simulink model "TPMCC_MCLV2_dsPIC33EP256MC506_V0_1"  (R2017a)
settings: Solver=FixedStepDiscrete  StartTime=0.0  StopTime=inf  FixedStep=Ts  RelTol=1e-3  EnableMultiTasking=on
values from neighbouring files (symbols this model uses):
  a = [1.0000   -0.5095]    [InitTPV0.m]
  b = [0.2452    0.2452]    [InitTPV0.m]
  Lignes = 250*4    (= 1000)    [InitTPV0.m]
  PWMmax = 3199    [InitTPV0.m]
  Tm = 0.5e-6    (= 5e-07)    [InitTPV0.m]
  TPWM = 1/FPWM    (= 5e-05)    [InitTPV0.m]
  Ts = 1e-4    (= 0.0001)    [InitTPV0.m]
  Vdc = 24    [InitTPV0.m]
undefined symbols (not defined in the file or in its folder): A4, A8, C5, C6, F1, P20, P24, P53, P54, P97, Pin, Timer
libraries: MCHP_Blockset x23, simulink x5
settings Model: Creator=rdelpoux  LastModifiedBy=rdelpoux
settings OptimizationCC: DefaultParameterBehavior=Inlined  DefaultUnderspecifiedDataType=single  BooleansAsBitfields=on  PassReuseOutputArgsAs=Individual arguments
settings DebuggingCC: ParameterOverflowMsg=warning  ParameterTunabilityLossMsg=error
settings HardwareCC: ProdBitPerInt=16  ProdBitPerPointer=16  ProdBitPerSizeT=16  ProdBitPerPtrDiffT=16  ProdLargestAtomicInteger=Integer  ProdLargestAtomicFloat=None  ProdWordSize=16  ProdHWDeviceType=Generic->Custom
settings ModelReferenceCC: ModelReferenceNumInstancesAllowed=Single
settings SFSimCC: MATLABDynamicMemAlloc=off
settings RTWCC: SystemTargetFile=MCHP_dsPIC_stf.tlc  TemplateMakefile=MCHP_dsPIC.tmf  Description=Microchip Embedded Target PIC24 dsPIC30 dsPIC33 (real-time)  GenerateReport=on  CustomSource=code.c  IncludeHyperlinkInReport=on  LaunchReport=on  GenerateTraceInfo=on  GenerateTraceReport=on  GenerateTraceReportSl=on  GenerateTraceReportSf=on  GenerateTraceReportEml=on
settings CodeAppCC: ForceParamTrailComments=on  IgnoreCustomStorageClasses=off  MaxIdLength=255  OperatorAnnotations=on  SimulinkDataObjDesc=on  SFDataObjDesc=on  MATLABFcnDesc=on  InsertBlockDesc=on  MATLABSourceComments=on
settings STFCustomTargetCC: TargetLibSuffix=_lib.a  MultiwordLength=256  IncludeMdlTerminateFcn=off  CombineOutputUpdateFcns=on  CombineSignalStateStructs=on  SuppressErrorStatus=on  ERTCustomFileBanners=on  SupportContinuousTime=off  RemoveResetFunc=on  MATLABClassNameForMDSCustomization=Simulink.SoftwareTarget.ERTCustomization  GRTInterface=off  SystemTargetFile=MCHP_dsPIC_stf.tlc
settings ERTTargetCC: TargetLibSuffix=_lib.a  ParMdlRefBuildCompliant=off  CompOptLevelCompliant=off  ConcurrentExecutionCompliant=off  IncludeMdlTerminateFcn=off  CombineSignalStateStructs=on  SuppressErrorStatus=on  ERTFirstTimeCompliant=off  SupportNonInlinedSFcns=on  ModelStepFunctionPrototypeControlCompliant=off  CPPClassGenCompliant=off  UseToolchainInfoCompliant=off  ExtModeStaticAllocSize=500  InlinedParameterPlacement=NonHierarchical  ERTSrcFileBannerTemplate=MCHP_dsPIC_code_template.cgt  ERTHdrFileBannerTemplate=MCHP_dsPIC_code_template.cgt  ERTDataSrcFileTemplate=MCHP_dsPIC_code_template.cgt  ERTDataHdrFileTemplate=MCHP_dsPIC_code_template.cgt  ERTCustomFileTemplate=MCHP_main.tlc

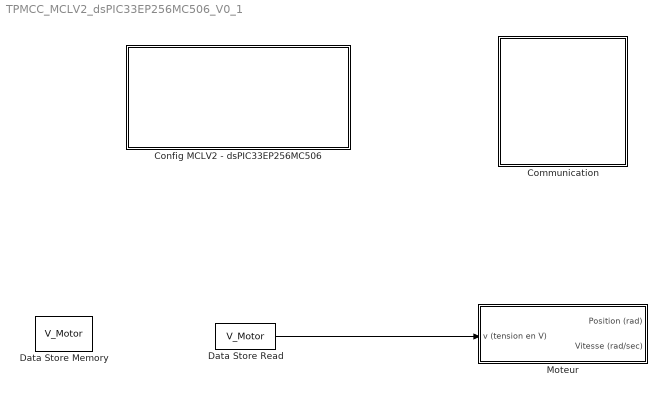
== system TPMCC_MCLV2_dsPIC33EP256MC506_V0_1 ==
  Communication : Subsystem
  "Config MCLV2 - dsPIC33EP256MC506 " : Subsystem
  Data Store Memory : DataStoreMemory  DataStoreName=V_Motor  ReadBeforeWriteMsg=warning  WriteAfterWriteMsg=warning  WriteAfterReadMsg=warning  ShowAdditionalParam=off  OutDataTypeStr=int16
  Data Store Read : DataStoreRead  DataStoreName=V_Motor  SampleTime=.01
  Moteur : Subsystem
  wires:
  Data Store Read/1 -> Moteur/1(v (tension en V))

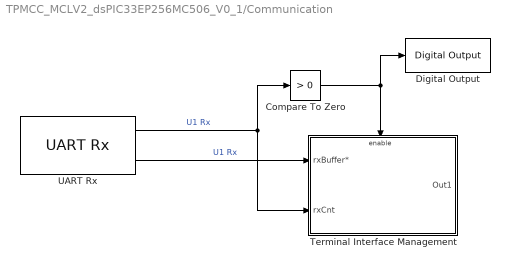
== system TPMCC_MCLV2_dsPIC33EP256MC506_V0_1/Communication ==
  Compare To Zero : simulink/Logic and Bit Operations/Compare To Zero  relop=>  OutDataTypeStr=boolean
  Digital Output : MCHP_Blockset/Digital IO/Digital Output  PORT=Dynamic Options  PORT_TXT="D   [ 5  6  8 ]"  PIN=[5]  PACK=off  SIMULTANEOUS=off  READPREVIOUS=off  ORDERING=None  SampleTime=-1  MCHP_MASTERLINK=TPMCC_MCLV2_dsPIC33EP256MC506_V0_1/Config MCLV2 - dsPIC33EP256MC506 /Microchip Master
      settings: SourceProductName=MPLAB® Device Blocks for Simulink®
  Terminal Interface Management : Subsystem
  UART Rx : MCHP_Blockset/BUS UART/UART Rx  UART_REF=1  Flag_Out=on  Rx_Size_popup=User defined  Rx_Size=100  S_Rx_Size=100  Split=Read all received char  SplitChar=13  OutputDefault_popup=Add one trailing 0  OutputDefault=-2  ORDERING=None  SampleTime=0.01  MCHP_MASTERLINK=TPMCC_MCLV2_dsPIC33EP256MC506_V0_1/Config MCLV2 - dsPIC33EP256MC506 /Microchip Master  MCHP_COMPILED_INFO="CompiledSampleTime= [0.01   0 ];CompiledInportDataTypes=[ ];CompiledInportDataWidth=[];"
      settings: SourceProductName=MPLAB® Device Blocks for Simulink®
  wires:
  UART Rx/2 -> Terminal Interface Management/1(rxBuffer*)  "U1 Rx"
  Compare To Zero/1 -> Digital Output/1, Terminal Interface Management/Enable
  UART Rx/1 -> Terminal Interface Management/2(rxCnt), Compare To Zero/1  "U1 Rx"

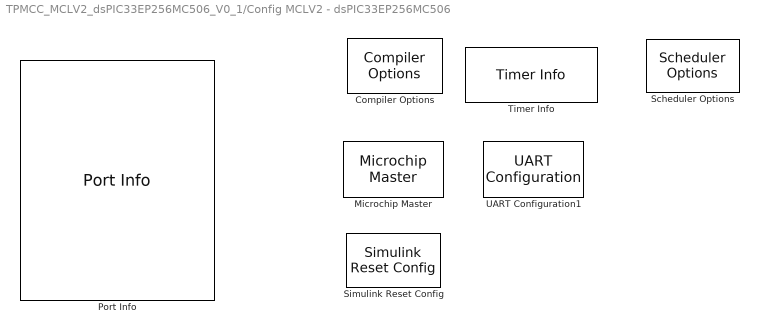
== system TPMCC_MCLV2_dsPIC33EP256MC506_V0_1/Config MCLV2 - dsPIC33EP256MC506  ==
  Compiler Options : MCHP_Blockset/System Configuration/Compiler Options  Priority=1  LATEST_CMPLR=on  COMP_LIST=xc16 - v1.34  COMP_LIST_TXT=xc16 - v1.34  USE_64BIT_DOUBLE=off  MCHP_MULTITHREAD_COMPILATION=on  UseCustom_LinkerScript=off  MCHP_MASTERLINK=TPMCC_MCLV2_dsPIC33EP256MC506_V0_1/Config MCLV2 - dsPIC33EP256MC506 /Microchip Master  OPTIMIZATION_LEVEL=3  MPLAB_LINKLIB=default  MPLAB_LINKLIB1=default  UNROLL_LOOPS=off  OMIT_FRAME_POINTER=off  PROCEDURAL_ABSTRACTION=off  MCONST=in code memory  MDATA=Use only memory below address 8192 (faster)  MSCALAR=Use only memory below address 8192 (faster)  MCODE=is less than 32768 (faster)  HEAP_SIZE=0  OMF=elf  DEBUG_INFO=on  AssemblyListing=off  ProduceHexOutput=on
      settings: SourceProductName=MPLAB® Device Blocks for Simulink®
  Microchip Master : MCHP_Blockset/System Configuration/Microchip Master  Priority=1  PICREF=33EP256MC506  TIMESTEP_REF="Timer  ( 0.0001s )"  BUSYFLAG=None  BUSYFLAG_TXT=None  PWRTEN=Not used  BOREN=Disable  BODENV=2.7V  BORV=Not used  FPWRT=128ms  DSBOREN=Enable ZPBOR during Deep Sleep Mode  DSLPBOR=Not used  MCLRE=Enabled  SMCLR=MCLR pin generates a normal system Reset  PMDL1WAY=Allow only one reconfiguration  RSTPRI=Device will obtain reset instruction from Primary flash  TEMP=Not used  SOSCSRC=Not used  SOSCSEL=Not used  IOL1WAY=Allow only one reconfiguration  ALTVREF=Not used  DISUVREG=Not used  DSSWEN=Not used  LPCFG=Not used  RTCBAT=Not used  VBTBOR=Not used  WUTSEL=Not used  POWERSAVE=off  FNOSC=Primary Oscillator (XT; HS; EC)  FPR=ECIO w/ PLL 16x  FOSFPR=HS3 w/PLL 16x  FOS=Primary Oscillator  FRANGE=High Range  OSCILLATOR_SELECT=Crystal / Ceramic resonator  OSCILLATOR_SELECT_spd=Crystal / Ceramic resonator  QUARTZ=8e6  QUARTZ_spd=8e6  POSCGAIN=2x gain setting  POSCBOOST=Boost the kick start of the oscillator  SOSCGAIN=2x gain setting  SOSCBOOST=Boost the kick start of the oscillator  ACTIV_PLL=on  ACTIV_PLL_spd=on  MIPS_DESIRED=64000000  MIPS_DESIRED_spd=64000000  FPLLMUL=Not used  FPLLIDIV=8x Divider  POSCFREQ=Not used  POSCMD=XT Crystal Oscillator Mode  POSCMOD=Primary osc disabled  MIPS=64 * 1e6  ACLKCON=Optimized for PWM resolution & ADC conversion speed  FPLLODIV=32x Divider  PLLKEN=Clock switch to PLL source will wait until the PLL lock signal is valid.  FCKSM=Clock switching is enabled;Fail-safe Clock Monitor is disabled  FCKSMEN=Sw Disabled; Mon Disabled  IESO=Start up with FRC; then switch  DSWDTPS=1:2^36  FWDTEN=Disable  FWDTWINSZ=Window size is 25%  FWPSA=1:512  FWPSA0=1:128  FWPSB=1:16  WDT=Disable  WDTPOST=1:32768  WDTPRE=1:128  WDTPS=1:1048576  WINDIS=Watchdog Timer in Non-Window mode  WWDTEN=Non-Window mode  DSWDTEN=Enable DSWDT during Deep Sleep Mode  DSWDTOSC=Select LPRC as DSWDT Reference clock  FPBDIV=Not used  FSOSCEN=Enable SOSC  LPRCSEL=Not used  OSCIOFCN=Not used  OSCIOFNC=OSC2 is clock output  LVRCFG=Not used  PLL_96MHZ=Not used  PLL96MHZ=Not used  PLLDIV=Not used  WDTCLK=Not used  WDTCMX=Not used  WDTWIN=WDT Window is 25% of WDT period  APL=Aux Flash Code protect is disabled  APLK=Aux Flash Write Protection or Code Protection is Enabled  AWRP=Auxiliary program memory is not write-protected  BSS=No Boot program Flash segment  BWP=Not used  BWRP=Boot Segment may be written  CP=Protection Disabled  EBS=No Boot EEPROM  ESS=No Segment Data EEPROM  GCP=General Segment Code protect is Disabled  GSS=General Segment Code protect is Disabled  GSS0=Not used  GSSK=General Segment Write Protection or Code Protection is Enabled  GWRP=General Segment may be written  PWP=Not used  RBS=No Boot RAM  RSS=No Secure RAM  SSS=No Secure Segment  SWRP=Secure segment may be written  WPCFG=Not used  WPDIS=Not used  WPEND=Not used  WPFP=Not used  ICESEL=Communicate on PGEC1/PGED1  ICS=Communicate on PGEC1 and PGED1  JTAGEN=Disable  COE=Not used  RES=Not used  DEBUG=Debugger is disabled  BACKBUG=Not used  BKBUG=Not used  ALTI2C=I2C mapped to SDA1/SCL1 pins  ALTI2C1=I2C1 mapped to SDA1/SCL1 pins  ALTI2C2=I2C2 mapped to SDA2/SCL2 pins  ALTQIO=QEA1; QEB1; INDX1 are selected as inputs to QEI1  ALTSS1=SS1A is selected as the I/O pin for SPI1  CMPPOL0=Hysteresis is applied to falling edge  CMPPOL1=Hysteresis is applied to falling edge  FCANIO=Not used  FETHIO=Default Ethernet I/O  FMIIEN=MII Enabled  FSRSSEL=Not used  FUSBIDIO=Controlled by the USB Module  FVBUSONIO=Not used  HPOL=PWM module high side output pins have active-high output polarity  HYST0=45 mV Hysteresis  HYST1=45 mV Hysteresis  I2C1SEL=Not used  LPOL=PWM module low side output pins have active-high output polarity  PWMPIN=PWM module pins controlled by PORT register at device Reset  RTCOSC=Not used  UPLLEN=USB PLL Disabled  UPLLIDIV=Not used  ATMOD8=Not used  ALTPMP=Not used  I2C2SEL=Not used  ALTADREF=Not used  ALTCVREF=Not used  PWMLOCK=PWM registers may be written without key sequence  MCHP_TIMER_REQUEST={Time Step}{TS}0:2:3:1:[]:6400;  MCHP_TIMER_RESULT=[1 6399.0000000000027 ]  MCHP_PLLRegisters="[5    222  16385     -1]"  MCHPVAR=MCHP.fcy.MIPS=64000000;MCHP.fcy.SYSCLK=64000000;MCHP.fcy.ADC=64000000;MCHP.fcy.Comparator=64000000;MCHP.fcy.I2C=64000000;MCHP.fcy.SPI=64000000;MCHP.fcy.UART=64000000;MCHP.fcy.Timers=64000000;MCHP.fcy.OC=64000000;MCHP.fcy.IC=64000000;MCHP.fcy.Ports=64000000;MCHP.fcy.QEI=64000000;MCHP.PowerSave=0;MCHP.TimeStepFactor=MCHP_Fun.Hex2num('3FEFFFFFFFFFFFFC');MCHP.TimeStep_Timer=1;MCHP.NTIMERS=5;MCHP.id.name='33EP256MC506';MCHP.id.N=reshape([33 256 506],1,3);MCHP.id.L=reshape({ 'EP','MC',''},1,3);MCHP.id.Arch=3;MCHP.periph.PPS.reg_RPINRx=reshape([-1 1 1 -1 -1 -1 1 -1 -1 -1 -1 -1 -1 -1 1 1 1 1 -1 -1 -1 -1 -1 -1 1 1 -1 -1 1 1 1 1 -1 -1 -1 -1 1 -1 1 -1 -1 -1 -1 -1 1 1 1 -1 -1 -1 -1 -1 1 -1 -1 -1 -1 -1 -1 -1 -1 -1 -1 -1 -1 -1 -1 -1 -1 -1 -1 -1 -1 -1 -1 1 -1 1 1 1],1,80);MCHP.PPS.dsPIC.RP=reshape([-1 -1 -1 -1 -1 -1 -1 -1 -1 -1 -1 -1 -1 -1 -1 -1 -1 -1 -1 -1 4 -1 -1 -1 -1 -1 -1 -1 -1 -1 -1 -1 -1 -1 -1 19 20 21 22 23 24 25 26 27 -1 -1 -1 -1 -1 -1 -1 -1 -1 -1 38 39 40 41 -1 -1 -1 -1 -1 -1 -1 -1 -1 -1 -1 -1 -1 -1 -1 -1 -1 -1 -1 -1 -1 -1 -1 -1 -1 -1 -1 -1 -1 -1 -1 -1 -1 -1 -1 -1 -1 -1 -1 81 -1 -1 -1 -1 -1 -1 -1 -1 -1 -1 -1 -1 -1 -1 -1 -1 -1 -1 -1 -1 102 -1 104],1,121);MCHP.PPS.dsPIC.RPI=reshape([-1 -1 -1 -1 -1 -1 -1 -1 -1 -1 -1 -1 -1 -1 -1 -1 -1 -1 -1 -1 -1 -1 -1 -1 8 9 -1 11 12 -1 -1 -1 16 17 18 -1 -1 -1 -1 -1 -1 -1 -1 -1 28 29 30 31 -1 -1 -1 35 36 37 -1 -1 -1 -1 42 -1 -1 -1 -1 -1 -1 -1 -1 -1 -1 -1 -1 -1 -1 -1 -1 -1 -1 -1 -1 -1 -1 -1 -1 -1 -1 -1 -1 -1 -1 -1 -1 -1 -1 -1 78 79 80 -1 -1 -1 -1 -1 -1 -1 -1 -1 -1 -1 -1 -1 -1 -1 -1 -1 -1 -1 -1 -1 -1 103 -1 105],1,122);MCHP.PPS.dsPIC.RPINR_list=reshape({ '1','INT1','INT2','INT3','INT4','T1CK','T2CK','T3CK','T4CK','T5CK','T6CK','T7CK','T8CK','T9CK','IC1','IC2','IC3','IC4','IC5','IC6','IC7','IC8','OCFA','OCFB','FLT1','FLT2','FLT3','FLT4','QEA1','QEB1','INDX1','HOME1','QEA2','QEB2','INDX2','HOME2','U1RX','U1CTS','U2RX','U2CTS','SDI1','SCK1_in','SS1_in','44','SDI2','SCK2_in','SS2_in','48','CSDIR','CSCK','COFS','52','C1RX','C2RX','U3RX','U3CTS','U4RX','U4CTS','SDI3','SCK3_in','SS3_in','62','SDI4','SCK4_in','SS4_in','66','IC9','IC10','IC11','IC12','IC13','IC14','IC15','IC16','OCFC','SYNCI1','SYNCI2','DTCMP1','DTCMP2','DTCMP3','DTCMP4','DTCMP5','DTCMP6','DTCMP7','FLT5','FLT6','FLT7','FLT8','89','SENT1','SENT2','92'},1,92);MCHP.PPS.dsPIC.RPOR_list=reshape({ '1','U1TX','U1RTS','U2TX','U2RTS','SDO1','SCK1_out','SS1_out','SDO2','SCK2_out','SS2_out','CSDO','CSCK','COFS','C1TX','C2TX','OC1','OC2','OC3','OC4','OC5','OC6','OC7','OC8','C1OUT','C2OUT','C3OUT','U3TX','U3RTS','U4TX','U4RTS','SDO3','SCK3_out','SS3_out','SDO4','SCK4_out','SS4_out','OC9','OC10','OC11','OC12','OC13','OC14','OC15','OC16','SYNCO1','SYNCO2','QEI1CCMP','QEI2CCMP','REFCLK','C4OUT','C5OUT','52','53','54','55','56','SENT1','SENT2'},1,59);MCHP.PPS.map_RPnR_RPORx=reshape([20 35 36 37 38 39 40 41 42 43 54 55 56 57 -1 97 -1 118 120],1,19);MCHP.Rx=reshape([13 15 21 -1 -1 58 -1 -1 -1 -1 -1 14 16 22 -1 -1 59 -1 -1 -1 -1 -1 -1 17 23 -1 -1 -1 -1 -1 -1 -1 -1 -1 18 35 -1 -1 -1 -1 -1 -1 -1 -1 33 32 36 -1 -1 -1 -1 -1 -1 -1 -1 -1 43 37 53 -1 -1 -1 -1 -1 -1 -1 -1 44 50 54 -1 -1 4 -1 -1 -1 -1 1 46 51 -1 -1 -1 5 -1 -1 -1 -1 31 48 52 42 -1 -1 6 -1 -1 -1 -1 34 49 55 -1 -1 -1 8 -1 -1 -1 -1 64 60 45 -1 -1 -1 -1 -1 -1 -1 -1 12 61 24 -1 -1 -1 -1 -1 -1 -1 -1 11 62 39 -1 27 -1 -1 -1 -1 -1 -1 -1 63 47 -1 28 -1 -1 -1 -1 -1 -1 -1 2 -1 -1 29 -1 -1 -1 -1 -1 -1 -1 3 40 -1 30 -1 -1 -1 -1 -1 -1],11,16);MCHP.ADC.ANtype=reshape([3 0],1,2);MCHP.ADC.ADCONx=reshape([47103 59391 40959 263 0 0],1,6);MCHP.ADC.ADCHS_0=reshape([40863 1799],1,2);MCHP.ADC.Flags=reshape([1 0],1,2);MCHP.ADC.Buffer=reshape([16 -1],1,2);MCHP.ADC.port=reshape([0 1 16 17 18 19 32 33 34 11 12 43 76 77 78 79 -1 -1 -1 -1 -1 -1 -1 -1 -1 -1 -1 -1 -1 -1 -1 -1 -1 -1 -1 -1 -1 -1 -1 -1 -1 -1 -1 -1 -1 -1 -1 -1 -1 -1 -1 -1 -1 -1 -1 -1 -1],1,57);MCHP.ADC.port_ALT=reshape([-1 -1 -1 -1],1,4);MCHP.ADC.port_VrefP=17;MCHP.ADC.port_VrefM=16;MCHP.ADC.port_AVdd=-1;MCHP.ADC.port_AVss=-1;MCHP.ADC.ADCDATA=reshape([0 0 0 0 0 0 0 0 0 0 0 0 0 0 0 0 0 0 0 0 0 0 0 0 0 0 0 0 0 0 0 0 0 0 0 0 0 0 0 0 0 0 0 0 0 0 0 0 0 0 0 0 0 0 0 0 0],1,57);MCHP.memory.RAM=32768;MCHP.memory.RAM_XBegin=4096;MCHP.memory.RAM_YBegin=20480;MCHP.memory.RAM_dma=reshape([-1 -1],1,2);MCHP.memory.FLASH_ECC=0;MCHP.DMA.Num=4;MCHP.DMA.CNTmax=16383;MCHP.QEI.QEICONx=reshape([49023 -1 -1 -1 -1 -1],1,6);MCHP.QEI.QEItype=1;MCHP.QEI.Port_QEI_INDX=reshape([-1 -1],1,2);MCHP.QEI.Port_QEI_QEA=reshape([-1 -1],1,2);MCHP.QEI.Port_QEI_QEB=reshape([-1 -1],1,2);MCHP.QEI.Port_QEI_UPDN=reshape([-1 -1],1,2);MCHP.INT.Port=reshape([23 32767 32767 -1 -1],1,5);MCHP.PWM_HS.Flags=reshape([3 1 0],1,3);MCHP.PWM.port_FLT=reshape([-1 -1 -1 34 43 -1 -1 -1 -1 -1 -1 -1 -1 -1 -1 -1 -1 -1 -1 -1 -1 -1 -1 -1 -1 -1 -1 -1 -1 -1 -1 -1 20],1,33);MCHP.PWM.PWMRef=-1;MCHP.PWM.Flag=0;MCHP.PWM.Port_PWM_l=reshape([31 -1 29 -1 27 -1 -1 -1 -1 -1 -1 -1 -1 -1 -1 -1 -1 -1 -1 -1 -1 -1 -1 -1],2,12);MCHP.PWM.Port_PWM_h=reshape([30 -1 28 -1 26 -1 -1 -1 -1 -1 -1 -1 -1 -1 -1 -1 -1 -1 -1 -1 -1 -1 -1 -1],2,12);MCHP.IC.Port=reshape([32767 32767 32767 32767 0 0 0 0 0 0 0 0 0 0 0 0],1,16);MCHP.IC.type=1;MCHP.OC.Port=reshape([32767 32767 32767 32767 0 0 0 0 0 0 0 0 0 0 0 0],1,16);MCHP.OC.type=1;MCHP.CN.Port=reshape([-1 -1 -1 -1 -1 -1 -1 -1 -1 -1 -1 -1 -1 -1 -1 -1 -1 -1 -1 -1 -1 -1 -1 -1 -1 -1 -1 -1 -1 -1 -1 -1 -1 -1 -1 -1 -1 -1 -1 -1 -1 -1 -1 -1 -1 -1 -1 -1 -1 -1 -1 -1 -1 -1 -1 -1 -1 -1 -1 -1 -1 -1 -1 -1 -1 -1 -1 -1 -1 -1 -1 -1 -1 -1 -1 -1 -1 -1 -1 -1 -1 -1 -1 -1 -1],1,85);MCHP.CN.PullUp=reshape([8083 65535 49151 352 61440 3 960 0 0 0 0],1,11);MCHP.CN.type=1;MCHP.CN.Flag_PullDown=1;MCHP.SPI.Refs=reshape([1 2 0 0 0 0],1,6);MCHP.SPI.SPIxCON1=8191;MCHP.SPI.SPIxCON2=57347;MCHP.SPI.Port_SDI=reshape([9 -1 -1 -1 -1 -1],1,6);MCHP.SPI.Port_SDO=reshape([4 -1 -1 -1 -1 -1],1,6);MCHP.SPI.Port_SCK=reshape([35 -1 -1 -1 -1 -1],1,6);MCHP.SPI.Port_SS=reshape([16 -1 -1 -1 -1 -1],1,6);MCHP.I2C.Refs=reshape([1 2 0 0 0],1,5);MCHP.I2C.I2CxCON=49151;MCHP.I2C.NewRegName=1;MCHP.I2C.Port_SDA=reshape([36 8 -1 -1 -1],1,5);MCHP.I2C.Port_SCL=reshape([37 20 -1 -1 -1],1,5);MCHP.I2C.Port_ASDA=reshape([25 21 -1 -1 -1],1,5);MCHP.I2C.Port_ASCL=reshape([24 22 -1 -1 -1],1,5);MCHP.I2C.Fuse_Port_SCL_SDA=reshape([3 1 4 1 -1 -1 -1 -1 -1 -1],2,5);MCHP.I2C.Fuse_Port_ASCL_ASDA=reshape([3 2 4 2 -1 -1 -1 -1 -1 -1],2,5);MCHP.PGA.Port_PGA1P=reshape([-1 -1 -1 -1],1,4);MCHP.PGA.Port_PGA1N=reshape([-1 -1 -1 -1],1,4);MCHP.PGA.Port_PGA2P=reshape([-1 -1 -1 -1],1,4);MCHP.PGA.Port_PGA2N=reshape([-1 -1 -1 -1],1,4);MCHP.PGA.Num=0;MCHP.HS_AnalogComparator.Port_CMP1=reshape([-1 -1 -1 -1],1,4);MCHP.HS_AnalogComparator.Port_CMP2=reshape([-1 -1 -1 -1],1,4);MCHP.HS_AnalogComparator.Port_CMP3=reshape([-1 -1 -1 -1],1,4);MCHP.HS_AnalogComparator.Port_CMP4=reshape([-1 -1 -1 -1],1,4);MCHP.HS_AnalogComparator.PORT_EXTREFx=reshape([-1 -1],1,2);MCHP.HS_AnalogComparator.Port_DACOUTx=reshape([-1 -1],1,2);MCHP.HS_AnalogComparator.Num=0;MCHP.Comp.Port_CVrefin=-1;MCHP.Comp.Port_CVref=-1;MCHP.Comp.Port_CVref1O=24;MCHP.Comp.Port_CVref2O=4;MCHP.Comp.Port_CxOUT=reshape([32767 32767 32767 32767 -1],1,5);MCHP.Comp.Port_OAxOUT=reshape([17 0 32 -1 -1],1,5);MCHP.Comp.Port_CxINP=reshape([18 1 34 32 -1],1,5);MCHP.Comp.Port_CxINM=reshape([19 43 -1 -1 16 76 -1 -1 33 77 -1 -1 33 -1 -1 -1 -1 -1 -1 -1],4,5);MCHP.Comp.nComp=reshape([4 0 0],1,3);MCHP.Comp.OpAmp=7;MCHP.Comp.CVRCON=reshape([17663 0],1,2);MCHP.CDAC.Port_DACx=reshape([-1 -1 -1],1,3);MCHP.CDAC.nCDAC=0;MCHP.UART.port_Rx=reshape([32767 32767 -1 -1 -1 -1],1,6);MCHP.UART.port_Tx=reshape([32767 32767 -1 -1 -1 -1],1,6);MCHP.UART.port_ARx=reshape([-1 -1],1,2);MCHP.UART.port_ATx=reshape([-1 -1],1,2);MCHP.UART.port_RTS=reshape([34 76 -1 -1 -1 -1],1,6);MCHP.UART.port_CTS=reshape([43 77 -1 -1 -1 -1],1,6);MCHP.UART.reg_UxMODE=reshape([48127 48127 -1 -1 -1 -1],1,6);MCHP.UART.reg_UxSTA=reshape([61439 61439 -1 -1 -1 -1],1,6);MCHP.modsrc.DOS_00794=1;MCHP.modsrc.DOS_00931=1;MCHP.modsrc.DOS_00932=1;MCHP.modsrc.DOS_00942=1;MCHP.modsrc.DOS_00938=1;MCHP.modsrc.DOS_00996=1;MCHP.modsrc.DOS_00997=1;MCHP.modsrc.DOS_00998=1;MCHP.modsrc.DOS_00209=0;MCHP.modsrc.DOS_01555_adc=0;MCHP.modsrc.DOS_01293=1;MCHP.modsrc.DOS_00828=0;MCHP.modsrc.DOS_01116=1;MCHP.modsrc.DOS_01017_RPORx=1;MCHP.modsrc.DOS_01017_RPINRx=1;MCHP.modsrc.DOS_01555_nvm_tsmc18_v2_16bit=0;MCHP.modsrc.DOS_00804=1;MCHP.modsrc.DOS_00826=1;MCHP.modsrc.DOS_01555_TLAK_PMDx=0;MCHP.modsrc.DOS_01555_TLAK_INT_=0;MCHP.modsrc.DOS_00933=1;MCHP.modsrc.DOS_01555=0;MCHP.modsrc.DOS_01555_ptg=0;MCHP.modsrc.DOS_00929=1;MCHP.modsrc.DOS_00958=1;MCHP.modsrc.DOS_01117_PORTx=1;MCHP.modsrc.DOS_00999=0;MCHP.modsrc.DOS_01198=1;MCHP.modsrc.DOS_01041=1;MCHP.modsrc.DOS_00892=1;MCHP.modsrc.DOS_01287_TLAC_PMDx=1;MCHP.modsrc.DOS_01287_TLAC_INT_=1;MCHP.modsrc.DOS_01424=1;MCHP.modsrc.DOS_01332=1;MCHP.modsrc.DOS_01441_i2c_upb_v1_16bit_TLAH=0;MCHP.modsrc.DOS_01482=0;MCHP.modsrc.DOS_02508c11=0;MCHP.modsrc.DOS_01468_PMBA_current_source=0;MCHP.modsrc.DOS_02291_PGA=0;MCHP.modsrc.DOS_01467_Comparator=0;MCHP.modsrc.DOS_01498_TLAY=0;MCHP.modsrc.DOS_02316_nvm_ctrl_v1_16bit=0;MCHP.modsrc.DOS_00993_PLL_120MHz=0;MCHP.modsrc.DOS_01577_cla_clc_upb_v1=0;MCHP.modsrc.DOS_01332_ptg_pc_v1=0;MCHP.modsrc.DOS_00958_pwm_TLAY=0;MCHP.modsrc.TLAY_IOPorts=0;MCHP.modsrc.DOS_00929q=0;MCHP.modsrc.DOS_02415_spi_v5=0;MCHP.modsrc.DOS_RPINRx_16bit_2=0;MCHP.modsrc.DOS_01497_TLAH_PMDx=0;MCHP.modsrc.DOS_02550_TLAL_INT=0;MCHP.modsrc.DOS_00958_pwm_TLAH=0;MCHP.modsrc.DOS_01287_TLAH_INT_=0;MCHP.modsrc.DOS_01113=0;MCHP.modsrc.DOS_01017_PMDx=0;MCHP.modsrc.DOS_00927=0;MCHP.modsrc.DOS_01080=0;MCHP.modsrc.DOS_00794_cpu_16bit_v3=0;MCHP.modsrc.DOS_02359a_sent_j2716_upb_v1=0;MCHP.modsrc.DOS_01520_wdt_dmt_upb_v1_16bit=0;MCHP.modsrc.DOS_02192_TLCD_PMDx=0;MCHP.modsrc.DOS_02192_TLCD_INT_=0;MCHP.modsrc.DOS_02192_cmp=0;MCHP.modsrc.DOS_00958_pwm_TLCD=0;MCHP.modsrc.DOS_02192_PORTx_TLCD=0;MCHP.modsrc.DOS_00936=0;MCHP.modsrc.DOS_00995=0;MCHP.modsrc.DOS_00546=0;MCHP.modsrc.DOS_00474=0;MCHP.modsrc.DOS_02481_WACJ_Config=0;MCHP.modsrc.DOS_02569_pfm_cache_ocp_v1=0;MCHP.modsrc.DOS_02819_pfm_ctrl_32bit_upb_v2=0;MCHP.modsrc.DOS_02674_wdt_upb_v1_32bit=0;MCHP.modsrc.DOS_01520_wdt_dmt_upb_v1=0;MCHP.modsrc.DOS_02869_icd_jtag_bvci_upb_v2=0;MCHP.modsrc.DOS_02823_WACJ_clk_cru_upb_v2=0;MCHP.modsrc.DOS_01423_RPINRx=0;MCHP.modsrc.DOS_02481_RPORx=0;MCHP.modsrc.DOS_02511_pwr_sib_upb_v1_32bit=0;MCHP.modsrc.DOS_02481_WACJ_int_evic_v3=0;MCHP.modsrc.DOS_01500_dma_bvci_v2=0;MCHP.modsrc.DOS_02141_tmr_classa_pb_v2=0;MCHP.modsrc.DOS_02815_tmr_classb_upb_v1=0;MCHP.modsrc.DOS_00740_icap_pb_v1=0;MCHP.modsrc.DOS_00749_ocmp_pb_v1=0;MCHP.modsrc.DOS_01441_i2c_upb_v1_32bit=0;MCHP.modsrc.DOS_01329_spi_pb_v2=0;MCHP.modsrc.DOS_02478_uart_irda_upb_v1_32bit=0;MCHP.modsrc.DOS_02514_dfm_strl_sst_upb_v1=0;MCHP.modsrc.DOS_01427_cmp_control_upb_v1_32bit=0;MCHP.modsrc.DOS_01445_dac_nbit__control_upb_v1_32bit=0;MCHP.modsrc.DOS_01461_afe_ctmu_con_upb_v1=0;MCHP.modsrc.DOS_02472_ppi_pmp16_upb_v1=0;MCHP.modsrc.DOS_02467_gpio_ports_upb_v1=0;MCHP.modsrc.DOS_02508_adc_sar_ctrl_upb_v1_PIC32MK=0;MCHP.modsrc.DOS_02813a_usb_otgcore_pb_v3=0;MCHP.modsrc.DOS_01261_tmr_rtcc_pb_v2=0;MCHP.modsrc.DOS_01475_lpwr_deep_sleep_ctrl_v2=0;MCHP.modsrc.DOS_EIP_00136_ssx_v1=0;MCHP.modsrc.DOS_01152_can_bvci_v1=0;MCHP.modsrc.DOS_02481_WACN_Config=0;MCHP.modsrc.DOS_02823_WACN_clk_cru_upb_v2=0;MCHP.modsrc.DOS_02481_WACN_int_evic_v3=0;MCHP.modsrc.DOS_03554_cmp_control_upb_v2_32bit=0;MCHP.modsrc.DOS_01577_cla_clc_upb_v1_32bit=0;MCHP.modsrc.DOS_03247_can_fd_upb_v2=0;MCHP.modsrc.DOS_02481_WACK_MC_Config=0;MCHP.modsrc.DOS_03247_can_fd_upb_v2_pic32mk=0;MCHP.modsrc.DOS_02481_WACJ_MC_Config=0;MCHP.modsrc.DOS_02481_WACJ_MC_int_evic_v3=0;MCHP.modsrc.DOS_01477_pwm_mc_upb_v1=0;MCHP.modsrc.DOS_01459_ptg_pc_upb_v1_SIC=0;MCHP.modsrc.DOS_01494_qei_32b_upb_v1=0;MCHP.modsrc.DOS_02481_WACN_MC_Config=0;MCHP.modsrc.DOS_02481_WACN_MC_int_evic_v3=0;MCHP.modsrc.DOS_02787_WACD_Config=0;MCHP.modsrc.DOS_00800_dac_4bit_ctrl_pb_v1=0;MCHP.modsrc.DOS_01539_icd_jtag_pb_v2=0;MCHP.modsrc.DOS_02823_clk_cru_upb_v2=0;MCHP.modsrc.DOS_01423_RPORx=0;MCHP.modsrc.DOS_02907_WACD_int_evic_v3=0;MCHP.modsrc.DOS_00734_uart_irda_pb_v1=0;MCHP.modsrc.DOS_00687_tmr_classa_pb_v1=0;MCHP.modsrc.DOS_00745_tmr_classb_pb_v1=0;MCHP.modsrc.DOS_02508_adc_sar_ctrl_upb_v1=0;MCHP.modsrc.DOS_00866_cmp_control_pb_v2=0;MCHP.modsrc.DOS_01114_eth_bvci_v1=0;MCHP.modsrc.DOS_02831_usb_clk_rst_v2=0;MCHP.modsrc.DOS_01643_pfm_cache_ahb_v2=0;MCHP.modsrc.DOS_EIP_00206r5_sqi_v2=0;MCHP.modsrc.DOS_EIP_00124_usb_hs_otgcore_v1=0;MCHP.modsrc.DOS_EIP_00218_math_rng_ahbs_v2=0;MCHP.modsrc.DOS_EIP_00109_ebi_v1=0;MCHP.modsrc.DOS_EIP_00158_crypto_v1=0;MCHP.clock.PBxDIV=-1;  MCHP_CRC=5664025  BTMODE=Not used  RES1=Not used  PLLSS=Not used  RES2=Not used  ALTCMPI=Not used  BOREN1=Not used  ALTRB6=Not used  RETCFG=Not used  DFMCY=Not used  BSS2=No Boot Segment  BSEN=No Boot Segment  CWRP=Configuration Segment may be written  CSS=No Protection (other than CWRP)  AIVTDIS=Disable Alternate Vector Table  BSLIM=Not used  WDTEN=Disable  BTSWP=BOOTSWP instruction is disabled  DBCC=No Cross Connection between DAC outputs  CTXT1=Not Assigned  CTXT2=Not Assigned  SEQNUM=Not used  nSEQNUM=Not used  BOREN0=Enabled  DMTIVT=Not used  DMTCNT=2^8 (256)  DMTEN=Dead Man Timer is Disabled and can be enabled by software  ON=Not used  USERID=Not used  RESERVED1=Not used  PGL1WAY=Allow only one reconfiguration  FPLLRNG=34-68 MHz Input  FPLLICLK=FRC is input to the System PLL  FPLLMULT=PLL Multiply by 128  UPLLFSEL=USB PLL input is 24 MHz  DMTINTV=Window/Interval value is 127/128 counter value  WDTSPGM=WDT stops during Flash programming  FDMTEN=Deadman Timer is disabled  TRCEN=Trace features in the CPU are enabled  BOOTISA=Boot code and Exception code is MIPS32  FECCCON=ECC and Dynamic ECC are disabled (ECCCON bits are writable)  EXTDDRSIZE=Not used  FSLEEP=Flash is powered down when the device is in Sleep mode  DBGPER=Allow CPU access to all permission regions  EJTAGBEN=Normal EJTAG functionality  TSEQ=Not used  CSEQ=Not used
      settings: SourceProductName=MPLAB® Device Blocks for Simulink®
  Port Info : MCHP_Blockset/System Info/Port Info  MCHP_MASTERLINK=TPMCC_MCLV2_dsPIC33EP256MC506_V0_1/Config MCLV2 - dsPIC33EP256MC506 /Microchip Master
      settings: SourceProductName=MPLAB® Device Blocks for Simulink®
  Scheduler Options : MCHP_Blockset/System Configuration/Scheduler Options  TaskOverloadBehaviour=Skip this task execution once  MCHP_MASTERLINK=UTester_33EP512MU810_CPUOverLoad/Microchip Master
      settings: SourceProductName=MPLAB® Device Blocks for Simulink®
  Simulink Reset Config : MCHP_Blockset/System Configuration/Simulink Reset Config  MCHP_MASTERLINK=0
      settings: SourceProductName=MPLAB® Device Blocks for Simulink®
  Timer Info : MCHP_Blockset/System Info/Timer Info  MCHP_MASTERLINK=TPMCC_MCLV2_dsPIC33EP256MC506_V0_1/Config MCLV2 - dsPIC33EP256MC506 /Microchip Master
      settings: SourceProductName=MPLAB® Device Blocks for Simulink®
  UART Configuration1 : MCHP_Blockset/BUS UART/UART Configuration  UART_REF=1  BAUD_Choice="115200         [-0.08%]"  BAUD_Choice_TXT="115200         [-0.08%]"  BAUD_Choice_IR="115200         [-0.79%]"  BAUD_Choice_IR_TXT=[]  BAUD_Custom=115200  ALT_IO=on  PIN_RX=C5 / P53 / Pin[37]  PIN_RX_TXT=C5 / P53 / Pin[37]  PIN_TX=F1 / P97 / Pin[59]  PIN_TX_TXT=F1 / P97 / Pin[59]  MCHP_PORT="{UART1  Rx}{U1RX}3:0:P53;{UART1  Tx}{U1TX}3:1:P97;"  MCHP_MASTERLINK=TPMCC_MCLV2_dsPIC33EP256MC506_V0_1/Config MCLV2 - dsPIC33EP256MC506 /Microchip Master  MCHP_COM_ExtPil=off  TX_IMPLEMENTATION=Circular Buffer  TX_IMPLEMENTATION_default=Circular Buffer  TX_INT_PRIORITY=6  TX_INT_WHEN=is empty  TX_INT_WHEN_default=is empty & last char is sent  TX_CIRCULAR_SIZE=2048  TX_DMA_CHANNEL="0   (Lowest Priority)"  TX_DMA_SIZE=[]  TX_TASK_PROTECTION=Delay tasks (default)  TX_INTERRUPT_PROTECTION=Do not send on conflict (default)  TX_INTERRUPT_PROTECTION_default=Do not send on conflict (default)  RX_IMPLEMENTATION=Simplest (4 bytes internal buffer only)  RX_IMPLEMENTATION_default=Circular Buffer  RX_INT_PRIORITY=1  RX_INT_WHEN=receive 1 character  RX_CIRCULAR_SIZE=2048  DuplexMode=Full duplex (default)  PIN_RX_Inv=off  PIN_TX_Inv=off  ParityBit=No parity (default)  StopBit=1 stop bit (default)  IRDA=off  FlowControl=None  PIN_CTS=A4 / P20 / Pin[33]  PIN_CTS_TXT=A4 / P20 / Pin[33]  PIN_RTS=A4 / P20 / Pin[33]  PIN_RTS_TXT=A4 / P20 / Pin[33]  InitSequence_chkbox=on  BAUD_Choice_InitSeq="115200         [-0.08%]"  BAUD_Choice_InitSeq_TXT="115200         [-0.08%]"  BAUD_Choice_IR_InitSeq="115200         [-0.79%]"  BAUD_Choice_IR_InitSeq_TXT=0  BAUD_Custom_InitSeq=0  InitSequence=['Init done' 10 13]
      settings: SourceProductName=MPLAB® Device Blocks for Simulink®

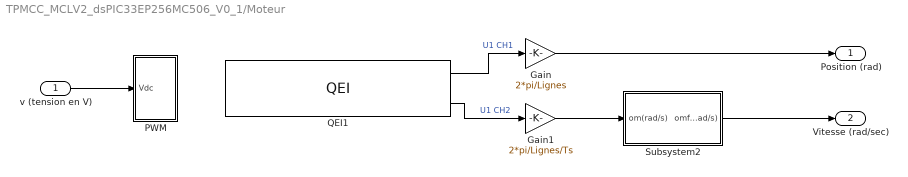
== system TPMCC_MCLV2_dsPIC33EP256MC506_V0_1/Moteur ==
  v (tension en V) : Inport
  Gain : Gain  Gain=2*pi/Lignes  OutDataTypeStr=fixdt(1,16,5)
  Gain1 : Gain  Gain=2*pi/Lignes/Ts  OutDataTypeStr=fixdt(1,16,5)  LockScale=on
  PWM : Subsystem
  QEI1 : MCHP_Blockset/QEI/QEI  QEI_REF=1  QEI_MODE=Quadrature Encoder  QEI_x2mode=off  QEI_PulseCountDir=Down  PIN_QEA=A8 / P24 / Pin[31]  PIN_QEA_TXT=A8 / P24 / Pin[31]  PIN_QEB=C6 / P54 / Pin[50]  PIN_QEB_TXT=C6 / P54 / Pin[50]  SWPAB=off  QEAPOL=off  QEBPOL=off  SampleTime=Ts  INDXxCNT_Output=is not an output  POSxCNT_Output=is a 16 bits unsigned block output  RESET_Input=off  PIMOD_mode=position is cyclique between user defined boundaries  PIMOD_modeB=Never reset position  PIMOD_reset=on next INDEX event  PIN_INDEX=A4 / P20 / Pin[33]  PIN_INDEX_TXT=A4 / P20 / Pin[33]  IMV=QEA = 1 and QEB = 0  IMV_x2=QEA = 1  PIN_HOME=A4 / P20 / Pin[33]  PIN_HOME_TXT=A4 / P20 / Pin[33]  QEIxLEC_GEC=[0 (Lignes-1)]  QEIxIC=0  PCIIRQ=off  IDXPOL=off  HOMPOL=on  VELxCNT_Output=is a 16 bits unsigned block output  INTxHLD_Output=is not an output  MaxPeriod=1e-2  FILTREN=off  QFDIV_popup=83.33 kHz  QFDIV_popup_TXT=83.33 kHz  FILTER_CutOffFreq=100e3  PIN_CCMP=A4 / P20 / Pin[33]  PIN_CCMP_TXT=A4 / P20 / Pin[33]  MCHP_PORT={QEI1 A}{QEA1}5:0:P24;{QEI1 B}{QEB1}5:0:P54;  MCHP_MASTERLINK=TPMCC_MCLV2_dsPIC33EP256MC506_V0_1/Config MCLV2 - dsPIC33EP256MC506 /Microchip Master  QEI_IntPri=5
      settings: SourceProductName=MPLAB® Device Blocks for Simulink®
  Subsystem2 : Subsystem
  Position (rad) : Outport
  Vitesse (rad/sec) : Outport  Port=2
  wires:
  QEI1/2 -> Gain1/1  "U1 CH2"
  Gain1/1 -> Subsystem2/1(om(rad/s))
  Gain/1 -> Position (rad)/1
  v (tension en V)/1 -> PWM/1(Vdc)
  Subsystem2/1(omf (rad/s)) -> Vitesse (rad/sec)/1
  QEI1/1 -> Gain/1  "U1 CH1"

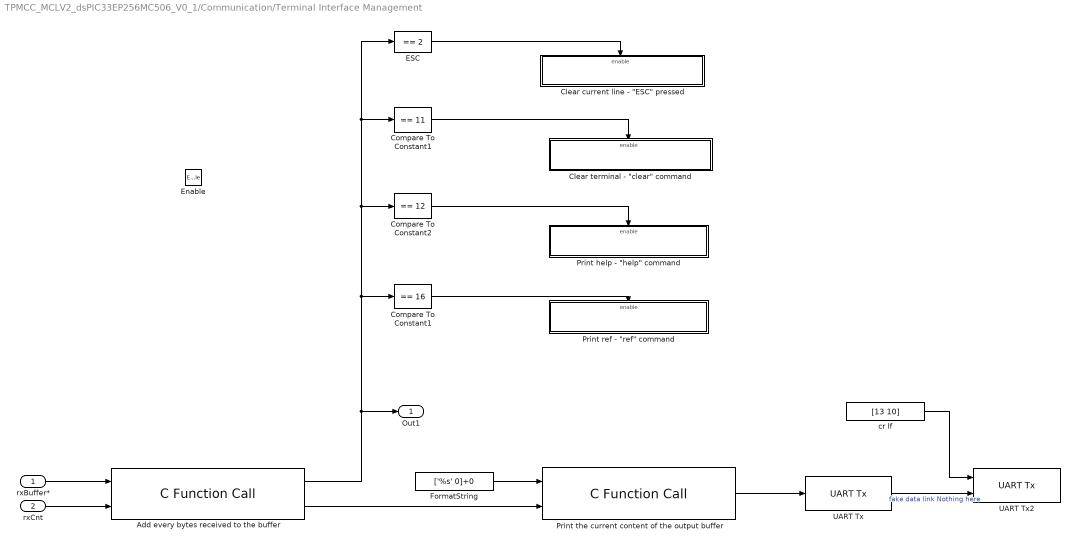
== system TPMCC_MCLV2_dsPIC33EP256MC506_V0_1/Communication/Terminal Interface Management ==
  rxBuffer* : Inport
  rxCnt : Inport  Port=2
  Enable : EnablePort
  Add every bytes received to the buffer : MCHP_Blockset/User Functions/C Function Call  Priority=0  ParseFilesChkbx=off  ListFunctions1=Custom Function  Function1=unsigned char addToBuffer( unsigned char outputBuffer[100], unsigned char *rxBuffer, unsigned int rxCnt)  AddHeaderDeclaration=off  Function1Type=when block is updated (default)  Fct1BlockIn=rxBuffer, rxCnt  FctReturnBlockOut=on  Fct1BlockOut=outputBuffer  DataCollected=0  ORDERING=None  SampleTime=-1  S_INPUT="[2  5]"  S_INPUT_Size="[-1  0  0  0  0  0  0  0  0  0  0  0  0  0  0  0  0  0  0  0]"  S_OUTPUT=[2]  S_OUTPUT_Size="[1  17   0   0   0   0   0   0   0   0]"  S_ListCustomDatatype=S.S_ListCustomDatatype={};  MCHP_CRC=1129636  MCHP_MASTERLINK=TPMCC_MCLV2_dsPIC33EP256MC506_V0_1/Config MCLV2 - dsPIC33EP256MC506 /Microchip Master  PinDigitalInput=[]  PinDigitalOutput=[]  PinAnalogInput=[]
      settings: SourceProductName=MPLAB® Device Blocks for Simulink®
  "Clear current line - \"ESC\" pressed" : Subsystem  Priority=1  TreatAsAtomicUnit=on
  "Clear terminal - \"clear\" command" : Subsystem  Priority=100
  Compare To Constant1 : simulink/Logic and Bit Operations/Compare To Constant  relop===  const=11  OutDataTypeStr=uint8
  Compare To Constant1 : simulink/Logic and Bit Operations/Compare To Constant  relop===  const=16  OutDataTypeStr=uint8
  Compare To Constant2 : simulink/Logic and Bit Operations/Compare To Constant  relop===  const=12  OutDataTypeStr=uint8
  ESC : simulink/Logic and Bit Operations/Compare To Constant  relop===  const=2  OutDataTypeStr=uint8
  "FormatString " : Constant  Priority=15  Value=['%s' 0]+0  OutDataTypeStr=uint8  LockScale=on
  "Print help - \"help\" command" : Subsystem  Priority=99
  "Print ref - \"ref\" command" : Subsystem  Priority=99
  Print the current content of the output buffer : MCHP_Blockset/User Functions/C Function Call  Priority=16  ParseFilesChkbx=off  ListFunctions1=Custom Function  Function1=void sprintf(unsigned char outputBuffer[100], const unsigned char* formatString, unsigned char* rxBuffer)  AddHeaderDeclaration=off  Function1Type=when block is updated (default)  Fct1BlockIn=formatString , rxBuffer  FctReturnBlockOut=off  Fct1BlockOut=outputBuffer  DataCollected=0  ORDERING=None  SampleTime=-1  S_INPUT="[2  5]"  S_INPUT_Size="[-1  0  0  0  0  0  0  0  0  0  0  0  0  0  0  0  0  0  0  0]"  S_OUTPUT=[2]  S_OUTPUT_Size="[1  17   0   0   0   0   0   0   0   0]"  S_ListCustomDatatype=S.S_ListCustomDatatype={};  MCHP_CRC=1157108  MCHP_MASTERLINK=TPMCC_MCLV2_dsPIC33EP256MC506_V0_1/Config MCLV2 - dsPIC33EP256MC506 /Microchip Master  PinDigitalInput=[]  PinDigitalOutput=[]  PinAnalogInput=[]
      settings: SourceProductName=MPLAB® Device Blocks for Simulink®
  UART Tx : MCHP_Blockset/BUS UART/UART Tx  Priority=17  UART_REF=1  ORDERING=Output  AllOrNothing=off  SampleTime=-1  MCHP_MASTERLINK=TPMCC_MCLV2_dsPIC33EP256MC506_V0_1/Config MCLV2 - dsPIC33EP256MC506 /Microchip Master  NSend_Input=off  UART_String=on  NSend_Output=off
      settings: SourceProductName=MPLAB® Device Blocks for Simulink®
  UART Tx2 : MCHP_Blockset/BUS UART/UART Tx  Priority=17  UART_REF=1  ORDERING=Input  AllOrNothing=off  SampleTime=-1  MCHP_MASTERLINK=TPMCC_MCLV2_dsPIC33EP256MC506_V0_1/Config MCLV2 - dsPIC33EP256MC506 /Microchip Master  NSend_Input=off  UART_String=on  NSend_Output=off
      settings: SourceProductName=MPLAB® Device Blocks for Simulink®
  cr lf : Constant  Priority=15  Value=[13 10]  OutDataTypeStr=uint8  LockScale=on
  Out1 : Outport
  wires:
  rxBuffer*/1 -> Add every bytes received to the buffer/1
  rxCnt/1 -> Add every bytes received to the buffer/2
  "FormatString "/1 -> Print the current content of the output buffer/1
  Print the current content of the output buffer/1 -> UART Tx/1
  Add every bytes received to the buffer/2 -> Print the current content of the output buffer/2
  Compare To Constant1/1 -> "Clear terminal - \"clear\" command"/Enable
  Compare To Constant2/1 -> "Print help - \"help\" command"/Enable
  ESC/1 -> "Clear current line - \"ESC\" pressed"/Enable
  Compare To Constant1/1 -> "Print ref - \"ref\" command"/Enable
  Add every bytes received to the buffer/1 -> Compare To Constant1/1, Compare To Constant2/1, ESC/1, Compare To Constant1/1, Out1/1
  cr lf/1 -> UART Tx2/1
  UART Tx/1 -> UART Tx2/2  "fake data link Nothing here"

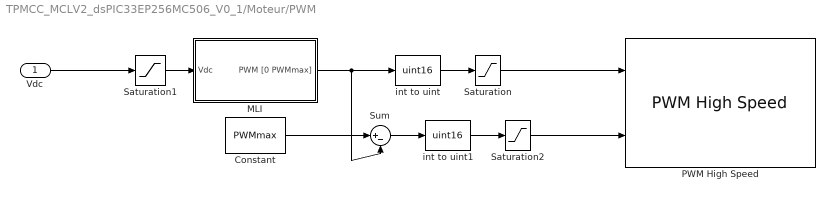
== system TPMCC_MCLV2_dsPIC33EP256MC506_V0_1/Moteur/PWM ==
  Vdc : Inport
  Constant : Constant  Value=PWMmax  OutDataTypeStr=uint16
  MLI : Subsystem
  PWM High Speed : MCHP_Blockset/PWM IO/PWM High Speed  pop1=[1]  chk1="[1  1  1  0  0]"  chkHL1="[1  1  0  1  1  1  1 ; 1  1  0  1  1  1  1]"  maxP1={ 'TPWM','0.001','0.001','0.001','0.001','0.001','0.001';'0.001','0.001','1e-06','0.001','0.001','0.001','0.001'}  InitP2={ 'TPWM','0.001','0.001','0.001','0.001','0.001','0.001';'0.001','0.001','0.001','0.001','0.001','0.001','0.001'}  chkP2="[0  1  0  1  1  1  1 ; 1  0  0  1  1  1  1]"  InitDC={ '50','50','50','50','50','50','50';'0.001','0.001','0.001','50','50','50','50'}  chkDC="[1  1  1  1  1  1  1 ; 0  0  0  1  1  1  1]"  InitPh={ '0','0','0','0.001','0.001','0.001','0.001';'0','0','0','0.001','0.001','0.001','0.001'}  chkPh="[0  0  0  1  1  1  1 ; 0  0  0  1  1  1  1]"  edSEvTrigx={ '0','-1','-1','-1','-1','-1','-1'}  chkSEvTrigx="[0  1  1  1  1  1  1]"  popFlt="[1  1  1  1  1  1  1]"  popFltPin="[24  25  20   4   4   4   4]"  popFltPinRp="[1  1  1  1  1  1  1]"  popFltActivH="[1  2  1  1  1  1  1]"  popFltForceH="[2  2  2  2  2  2  2]"  popFltForceL="[1  1  1  1  1  1  1]"  chkFltBlkOut="[0  0  0  0  0  0  0]"  popIndepFaultMode="[1  1  1  1  1  1  1]"  popCurEnabled="[1  1  1  1  1  1  1]"  popCurPin="[4  31   4   4   4   4   4]"  popCurActiveH="[1  1  1  1  1  1  1]"  popCurForceH="[2  1  2  1  1  1  1]"  popCurForceL="[2  1  2  1  1  1  1]"  ChkCurBlkOut="[1  0  0  0  0  0  0]"  ChkCurBlkOutTime="[1  0  1  0  0  0  0]"  popBLANKSEL="[1  1  1  1  1  1  1]"  popBPHHBPHL="[1  1  1  1  1  1  1]"  popBPLHBPLL="[1  1  1  1  1  1  1]"  popFLTLEBEN_CLLEBEN="[1  1  1  1  1  1  1]"  popPHR_PHF="[2  1  1  1  1  1  1]"  popPLR_PLF="[3  1  1  1  1  1  1]"  edLEB={ '100e-9','50e-9','150e-9','50e-9','50e-9','50e-9','50e-9'}  popDT="[1  1  1  3  3  3  3]"  edDTRx={ '0.02','1e-05','0.001','1e-05','1e-05','1e-05','1e-05'}  edAltDTRx={ 'Tm','Tm','Tm','1e-05','1e-05','1e-05','1e-05'}  S_INPUT="[5  5  5]"  S_INPUT_Size="[1  1  1]"  S_OUTPUT=[]  S_OUTPUT_Size=[]  S_DWORK_Type=[]  S_DWORK_Size=[]  ADC_VARTRIG={PWM Primary Special Event Trigger;6}  SampleTime=-1  ORDERING=None  MCHP_PORT={PWM1H}{PWM1H}4:4:B14;{PWM1L}{PWM1L}4:4:B15;{PWM2H}{PWM2H}4:4:B12;{PWM2L}{PWM2L}4:4:B13;  MCHP_MASTERLINK=TPMCC_MCLV2_dsPIC33EP256MC506_V0/Config MCLV2 - dsPIC33EP256MC506 /Microchip Master  MCHP_VERSION=v3.39
      settings: SourceProductName=MPLAB® Device Blocks for Simulink®
  Saturation : Saturate  UpperLimit=PWMmax  LowerLimit=round( (Tm/TPWM) *PWMmax )
  Saturation1 : Saturate  UpperLimit=Vdc  LowerLimit=-Vdc
  Saturation2 : Saturate  UpperLimit=PWMmax  LowerLimit=round( (Tm/TPWM) *PWMmax )
  Sum : Sum  Inputs=|+-
  int to uint : DataTypeConversion  OutDataTypeStr=uint16  ConvertRealWorld=Stored Integer (SI)
  int to uint1 : DataTypeConversion  OutDataTypeStr=uint16  ConvertRealWorld=Stored Integer (SI)
  wires:
  Vdc/1 -> Saturation1/1
  MLI/1(PWM [0 PWMmax]) -> Sum/2, int to uint/1
  int to uint/1 -> Saturation/1
  Saturation/1 -> PWM High Speed/1
  Saturation1/1 -> MLI/1(Vdc)
  int to uint1/1 -> Saturation2/1
  Saturation2/1 -> PWM High Speed/2
  Sum/1 -> int to uint1/1
  Constant/1 -> Sum/1

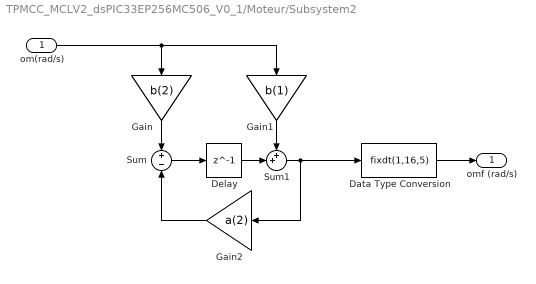
== system TPMCC_MCLV2_dsPIC33EP256MC506_V0_1/Moteur/Subsystem2 ==
  om(rad/s) : Inport
  Data Type Conversion : DataTypeConversion  OutMin=[-500]  OutMax=[500]  OutDataTypeStr=fixdt(1,16,5)
  Delay : Delay  DelayLength=1  InitialCondition=0  SampleTime=Ts
  Gain : Gain  Gain=b(2)  ParamDataTypeStr=fixdt(1,16,21)  OutMin=[b(2)*-500]  OutMax=[b(2)*500]  OutDataTypeStr=fixdt(1,16,12)
  Gain1 : Gain  Gain=b(1)  ParamDataTypeStr=fixdt(1,16,21)  OutMin=[b(1)*-500]  OutMax=[b(1)*500]  OutDataTypeStr=fixdt(1,16,12)
  Gain2 : Gain  Gain=a(2)  ParamDataTypeStr=fixdt(1,16,15)  OutMin=[-a(2)*-500]  OutMax=[-a(2)*500]  OutDataTypeStr=fixdt(1,16,6)
  Sum : Sum  Inputs=+|-
  Sum1 : Sum  Inputs=++|
  omf (rad/s) : Outport
  wires:
  Data Type Conversion/1 -> omf (rad/s)/1
  Delay/1 -> Sum1/2
  Sum1/1 -> Gain2/1, Data Type Conversion/1
  Gain2/1 -> Sum/2
  Gain1/1 -> Sum1/1
  Gain/1 -> Sum/1
  Sum/1 -> Delay/1
  om(rad/s)/1 -> Gain/1, Gain1/1

== system TPMCC_MCLV2_dsPIC33EP256MC506_V0_1/Communication/Terminal Interface Management/Clear current line - "ESC" pressed ==
  Enable : EnablePort
  Clear current line : Subsystem  Priority=0  TreatAsAtomicUnit=on

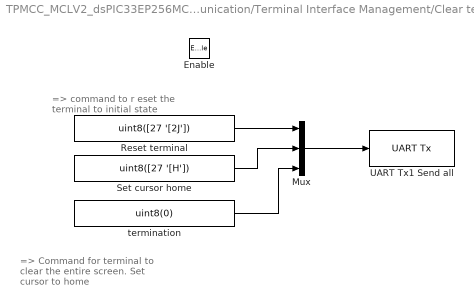
== system TPMCC_MCLV2_dsPIC33EP256MC506_V0_1/Communication/Terminal Interface Management/Clear terminal - "clear" command ==
  note: => command to r eset the terminal to initial state
  note: => Command for terminal to clear the entire screen. Set cursor to home
  Enable : EnablePort
  Mux : Mux  Inputs=3
  Reset terminal : Constant  Priority=0  Value=uint8([27 '[2J'])  LockScale=on
  Set cursor home : Constant  Priority=0  Value=uint8([27 '[H'])  LockScale=on
  UART Tx1 Send all : MCHP_Blockset/BUS UART/UART Tx  UART_REF=1  ORDERING=None  AllOrNothing=off  SampleTime=-1  MCHP_MASTERLINK=TPMCC_MCLV2_dsPIC33EP256MC506_V0_1/Config MCLV2 - dsPIC33EP256MC506 /Microchip Master  NSend_Input=off  UART_String=off  NSend_Output=off
      settings: SourceProductName=MPLAB® Device Blocks for Simulink®
  termination : Constant  Priority=0  Value=uint8(0)  LockScale=on
  wires:
  Reset terminal/1 -> Mux/1
  Set cursor home/1 -> Mux/2
  Mux/1 -> UART Tx1 Send all/1
  termination/1 -> Mux/3

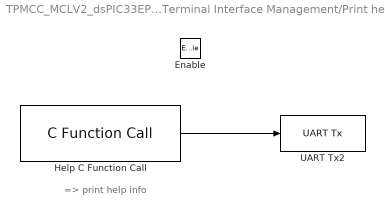
== system TPMCC_MCLV2_dsPIC33EP256MC506_V0_1/Communication/Terminal Interface Management/Print help - "help" command ==
  note: => print help info
  Enable : EnablePort
  Help C Function Call : MCHP_Blockset/User Functions/C Function Call  Priority=0  ParseFilesChkbx=off  ListFunctions1=Custom Function  Function1=void printHelp(unsigned char str[5000])  AddHeaderDeclaration=off  Function1Type=when block is updated (default)  FctReturnBlockOut=off  Fct1BlockOut=str  DataCollected=0  ORDERING=None  SampleTime=-1  S_INPUT="[2  5]"  S_INPUT_Size="[-1  0  0  0  0  0  0  0  0  0  0  0  0  0  0  0  0  0  0  0]"  S_OUTPUT=[2]  S_OUTPUT_Size="[1  17   0   0   0   0   0   0   0   0]"  S_ListCustomDatatype=S.S_ListCustomDatatype={};  MCHP_CRC=805532  MCHP_MASTERLINK=TPMCC_MCLV2_dsPIC33EP256MC506_V0_1/Config MCLV2 - dsPIC33EP256MC506 /Microchip Master  PinDigitalInput=[]  PinDigitalOutput=[]  PinAnalogInput=[]
      settings: SourceProductName=MPLAB® Device Blocks for Simulink®
  UART Tx2 : MCHP_Blockset/BUS UART/UART Tx  UART_REF=1  ORDERING=None  AllOrNothing=off  SampleTime=-1  MCHP_MASTERLINK=TPMCC_MCLV2_dsPIC33EP256MC506_V0_1/Config MCLV2 - dsPIC33EP256MC506 /Microchip Master  NSend_Input=off  UART_String=on  NSend_Output=off
      settings: SourceProductName=MPLAB® Device Blocks for Simulink®
  wires:
  Help C Function Call/1 -> UART Tx2/1

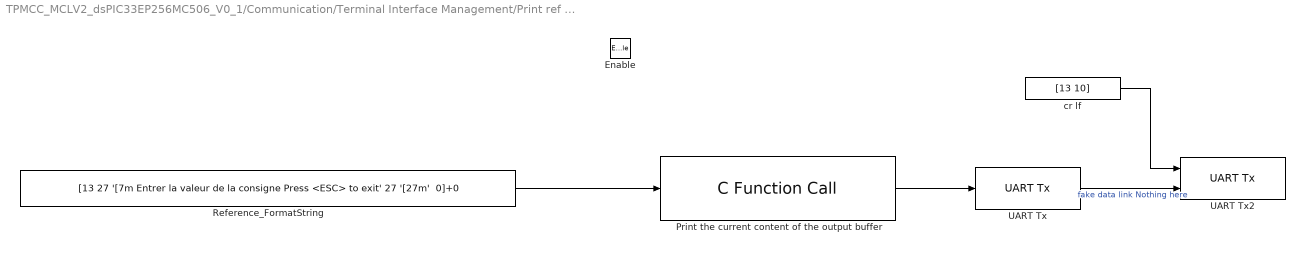
== system TPMCC_MCLV2_dsPIC33EP256MC506_V0_1/Communication/Terminal Interface Management/Print ref - "ref" command ==
  Enable : EnablePort
  Print the current content of the output buffer : MCHP_Blockset/User Functions/C Function Call  Priority=16  ParseFilesChkbx=off  ListFunctions1=Custom Function  Function1=void sprintf(unsigned char outputBuffer[100], const char* formatString)  AddHeaderDeclaration=off  Function1Type=when block is updated (default)  Fct1BlockIn=formatString  FctReturnBlockOut=off  Fct1BlockOut=outputBuffer  DataCollected=0  ORDERING=None  SampleTime=-1  S_INPUT="[2  5]"  S_INPUT_Size="[-1  0  0  0  0  0  0  0  0  0  0  0  0  0  0  0  0  0  0  0]"  S_OUTPUT=[2]  S_OUTPUT_Size="[1  17   0   0   0   0   0   0   0   0]"  S_ListCustomDatatype=S.S_ListCustomDatatype={};  MCHP_CRC=1036052  MCHP_MASTERLINK=TPMCC_MCLV2_dsPIC33EP256MC506_V0_1/Config MCLV2 - dsPIC33EP256MC506 /Microchip Master  PinDigitalInput=[]  PinDigitalOutput=[]  PinAnalogInput=[]
      settings: SourceProductName=MPLAB® Device Blocks for Simulink®
  Reference_FormatString : Constant  Value="[13 27 '[7m Entrer la valeur de la consigne Press <ESC> to exit' 27 '[27m'  0]+0"  OutDataTypeStr=int8  SampleTime=-1  LockScale=on
  UART Tx : MCHP_Blockset/BUS UART/UART Tx  Priority=17  UART_REF=1  ORDERING=Output  AllOrNothing=off  SampleTime=-1  MCHP_MASTERLINK=TPMCC_MCLV2_dsPIC33EP256MC506_V0_1/Config MCLV2 - dsPIC33EP256MC506 /Microchip Master  NSend_Input=off  UART_String=on  NSend_Output=off
      settings: SourceProductName=MPLAB® Device Blocks for Simulink®
  UART Tx2 : MCHP_Blockset/BUS UART/UART Tx  Priority=17  UART_REF=1  ORDERING=Input  AllOrNothing=off  SampleTime=-1  MCHP_MASTERLINK=TPMCC_MCLV2_dsPIC33EP256MC506_V0_1/Config MCLV2 - dsPIC33EP256MC506 /Microchip Master  NSend_Input=off  UART_String=on  NSend_Output=off
      settings: SourceProductName=MPLAB® Device Blocks for Simulink®
  cr lf : Constant  Priority=15  Value=[13 10]  OutDataTypeStr=uint8  LockScale=on
  wires:
  Print the current content of the output buffer/1 -> UART Tx/1
  Reference_FormatString/1 -> Print the current content of the output buffer/1
  UART Tx/1 -> UART Tx2/2  "fake data link Nothing here"
  cr lf/1 -> UART Tx2/1

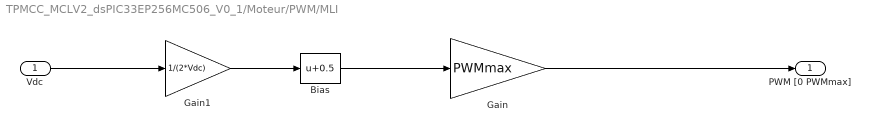
== system TPMCC_MCLV2_dsPIC33EP256MC506_V0_1/Moteur/PWM/MLI ==
  Vdc : Inport
  Bias : Bias  Bias=0.5
  Gain : Gain  Gain=PWMmax  OutDataTypeStr=uint16
  Gain1 : Gain  Gain=1/(2*Vdc)  OutDataTypeStr=fixdt(1,16,14)  SaturateOnIntegerOverflow=on
  PWM [0 PWMmax] : Outport
  wires:
  Gain/1 -> PWM [0 PWMmax]/1
  Vdc/1 -> Gain1/1
  Gain1/1 -> Bias/1
  Bias/1 -> Gain/1

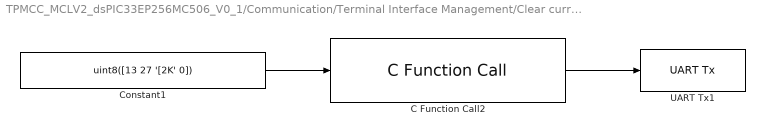
== system TPMCC_MCLV2_dsPIC33EP256MC506_V0_1/Communication/Terminal Interface Management/Clear current line - "ESC" pressed/Clear current line ==
  C Function Call2 : MCHP_Blockset/User Functions/C Function Call  ParseFilesChkbx=off  ListFunctions1=Custom Function  Function1=void sprintf(unsigned char outputBuffer[100], const unsigned char* formatString)  AddHeaderDeclaration=off  Function1Type=when block is updated (default)  Fct1BlockIn=formatString  FctReturnBlockOut=off  Fct1BlockOut=outputBuffer  DataCollected=0  ORDERING=None  SampleTime=-1  S_INPUT="[2  5]"  S_INPUT_Size="[-1  0  0  0  0  0  0  0  0  0  0  0  0  0  0  0  0  0  0  0]"  S_OUTPUT=[2]  S_OUTPUT_Size="[1  17   0   0   0   0   0   0   0   0]"  S_ListCustomDatatype=S.S_ListCustomDatatype={};  MCHP_CRC=1061045  MCHP_MASTERLINK=TPMCC_MCLV2_dsPIC33EP256MC506_V0_1/Config MCLV2 - dsPIC33EP256MC506 /Microchip Master  PinDigitalInput=[]  PinDigitalOutput=[]  PinAnalogInput=[]
      settings: SourceProductName=MPLAB® Device Blocks for Simulink®
  Constant1 : Constant  Value=uint8([13 27 '[2K' 0])  OutDataTypeStr=uint8  LockScale=on
  UART Tx1 : MCHP_Blockset/BUS UART/UART Tx  UART_REF=1  ORDERING=None  AllOrNothing=off  SampleTime=-1  MCHP_MASTERLINK=TPMCC_MCLV2_dsPIC33EP256MC506_V0_1/Config MCLV2 - dsPIC33EP256MC506 /Microchip Master  NSend_Input=off  UART_String=on  NSend_Output=off
      settings: SourceProductName=MPLAB® Device Blocks for Simulink®
  wires:
  Constant1/1 -> C Function Call2/1
  C Function Call2/1 -> UART Tx1/1
